simulink model "sim"  (R2018b)
settings: Solver=VariableStepAuto  StartTime=0.0  StopTime=10  RelTol=1e-3
values from neighbouring files (symbols this model uses):
  Force = 16    [variables.m]
  g = -9.81    [variables.m]
  m = 0.05    [variables.m]
  vChute = -20    [variables.m]
settings Model: Creator=diktux  LastModifiedBy=diktux

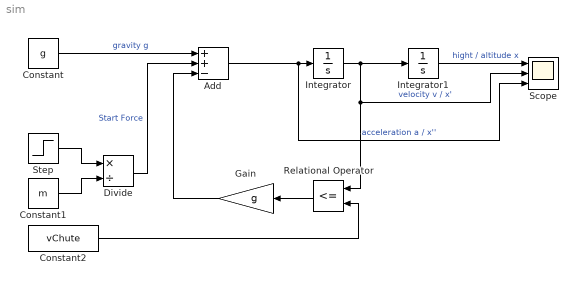
== system sim ==
  Add : Sum  Inputs=++-
  Constant : Constant  Value=g
  Constant1 : Constant  Value=m
  Constant2 : Constant  Value=vChute
  Divide : Product  Inputs=*/
  Gain : Gain  Gain=g
  Integrator : Integrator
  Integrator1 : Integrator
  Relational Operator : RelationalOperator  Operator=<=  OutDataTypeStr=boolean  RndMeth=Simplest
  Scope : Scope  NumInputPorts=3
  Step : Step  Time=0.15  Before=Force  After=0  SampleTime=0
  wires:
  Integrator/1 -> Scope/2, Relational Operator/1, Integrator1/1  "velocity v / x'"
  Integrator1/1 -> Scope/1  "hight / altitude x"
  Add/1 -> Scope/3, Integrator/1  "acceleration a / x''"
  Constant1/1 -> Divide/2
  Step/1 -> Divide/1
  Divide/1 -> Add/2  "Start Force"
  Constant/1 -> Add/1  "gravity g"
  Constant2/1 -> Relational Operator/2
  Relational Operator/1 -> Gain/1
  Gain/1 -> Add/3
